simulink model "ModelWithApproximation_20210821T210314460"  (R2020a)
settings: Solver=FixedStepAuto  StartTime=0.0  StopTime=size(InputValues_20210821T203440345,1) - 1  FixedStep=1  RelTol=1e-3
model workspace (MAT data in the model file):
  InputValues_20210821T203440345 = [-1 -0.9921875 -0.984375 -0.9765625 -0.96875 -0.9609375 -0.953125 -0.9453125 -0.9375 -0.9296875 -0.921875 -0.9140625 ... (256 elements, 256x1)]
undefined symbols (not defined in the file or in its folder): FunctionApproximation
libraries: simulink x1
settings Model: OrderedModelArguments=off  Creator=Mahsa  LastModifiedBy=Mahsa
settings DebuggingCC: IntegerOverflowMsg=none  ParameterOverflowMsg=none  ParameterPrecisionLossMsg=none  IntegerSaturationMsg=none

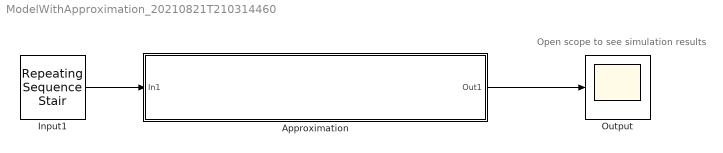
== system ModelWithApproximation_20210821T210314460 ==
  note: Open scope to see simulation results
  Approximation : Subsystem  Description=This block was created using function approximation.  Variant=on  mask(Function Approximation Solution){variantTag=119b4c483346d2625863553620acd5dc80d8d358, createdBy=FunctionApproximation, currentActive=Approximate, nApproximates=1, createdOn=20210821T210309766, matlabVersion={"Name":"MATLAB","Version":"9.8","Release":"(R2020a)","Date":"18-Nov-2019"}, functionVersion=Approximate, problemStruct={"FunctionToApproximate":"@(x)tanh(x)","InputTypes":"numerictype(1,8,7)","InputLowerBounds":"-1","InputUpperBounds":"0.9921875","OutputType":"numerictype(1,8,7)","Options":{"WordLengths":"[8]","BreakpointSpecification":"EvenSpacing","AbsTol":"0.0078125","RelTol":"0.0078125","AllowUpdateDiagram":"1","Display":"1","Interpolation":"Linear","SaturateToOutputType":"0","MaxTime":"Inf","MaxMemoryUsage":"80000000","MemoryUnits":"bits","OnCurveTableValues":"0","AUTOSARCompliant":"0","UseParallel":"0"},"FunctionToReplace":"","InputFunctionType":"SpecialFunctionHandle","StorageTypes":[],"DependentVariables":[]}, compareData={"Breakpoints":[[-1,-0.9921875,-0.984375,-0.9765625,-0.96875,-0.9609375,-0.953125,-0.9453125,-0.9375,-0.9296875,-0.921875,-0.9140625,-0.90625,-0.8984375,-0.890625,-0.8828125,-0.875,-0.8671875,-0.859375,-0.8515625,-0.84375,-0.8359375,-0.828125,-0.8203125,-0.8125,-0.8046875,-0.796875,-0.7890625,-0.78125,-0.7734375,-0.765625,-0.7578125,-0.75,-0.7421875,-0.734375,-0.7265625,-0.71875,-0.7109375,-0.703125,-0.6953125,-0.6875,-0.6796875,-0.671875,-0.6640625,-0.65625,-0.6484375,-0.640625,-0.6328125,-0.625,-0.6171875,-0.609375,-0.6015625,-0.59375,-0.5859375,-0.578125,-0.5703125,-0.5625,-0.5546875,-0.546875,-0.5390625,-0.53125,-0.5234375,-0.515625,-0.5078125,-0.5,-0.4921875,-0.484375,-0.4765625,-0.46875,-0.4609375,-0.453125,-0.4453125,-0.4375,-0.4296875,-0.421875,-0.4140625,-0.40625,-0.3984375,-0.390625,-0.3828125,-0.375,-0.3671875,-0.359375,-0.3515625,-0.34375,-0.3359375,-0.328125,-0.3203125,-0.3125,-0.3046875,-0.296875,-0.2890625,-0.28125,-0.2734375,-0.265625,-0.2578125,-0.25,-0.2421875,-0.234375,-0.2265625,-0.21875,-0.2109375,-0.203125,-0.1953125,-0.1875,-0.1796875,-0.171875,-0.1640625,-0.15625,-0.1484375,-0.140625,-0.1328125,-0.125,-0.1171875,-0.109375,-0.1015625,-0.09375,-0.0859375,-0.078125,-0.0703125,-0.0625,-0.0546875,-0.046875,-0.0390625,-0.03125,-0.0234375,-0.015625,-0.0078125,0,0.0078125,0.015625,0.0234375,0.03125,0.0390625,0.046875,0.0546875,0.0625,0.0703125,0.078125,0.0859375,0.09375,0.1015625,0.109375,0.1171875,0.125,0.1328125,0.140625,0.1484375,0.15625,0.1640625,0.171875,0.1796875,0.1875,0.1953125,0.203125,0.2109375,0.21875,0.2265625,0.234375,0.2421875,0.25,0.2578125,0.265625,0.2734375,0.28125,0.2890625,0.296875,0.3046875,0.3125,0.3203125,0.328125,0.3359375,0.34375,0.3515625,0.359375,0.3671875,0.375,0.3828125,0.390625,0.3984375,0.40625,0.4140625,0.421875,0.4296875,0.4375,0.4453125,0.453125,0.4609375,0.46875,0.4765625,0.484375,0.4921875,0.5,0.5078125,0.515625,0.5234375,0.53125,0.5390625,0.546875,0.5546875,0.5625,0.5703125,0.578125,0.5859375,0.59375,0.6015625,0.609375,0.6171875,0.625,0.6328125,0.640625,0.6484375,0.65625,0.6640625,0.671875,0.6796875,0.6875,0.6953125,0.703125,0.7109375,0.71875,0.7265625,0.734375,0.7421875,0.75,0.7578125,0.765625,0.7734375,0.78125,0.7890625,0.796875,0.8046875,0.8125,0.8203125,0.828125,0.8359375,0.84375,0.8515625,0.859375,0.8671875,0.875,0.8828125,0.890625,0.8984375,0.90625,0.9140625,0.921875,0.9296875,0.9375,0.9453125,0.953125,0.9609375,0.96875,0.9765625,0.984375,0.9921875]],"Original":[-0.76159415595576485,-0.75829353501905861,-0.75495357496368154,-0.7515739832958932,-0.74815447032973548,-0.74469474935641866,-0.74119453681672176,-0.73765355247636877,-0.73407151960434158,-0.73044816515408639,-0.72678321994756123,-0.7230764188620713,-0.71932750101983345,-0.71553620998020728,-0.71170229393451878,-0.70782550590340865,-0.70390560393662116,-0.69994235131514981,-0.69593551675565146,-0.69188487461702919,-0.68779020510908528,-0.68365129450313655,-0.67946793534447858,-0.67523992666657839,-0.67096707420687374,-0.66664919062404671,-0.66228609571663366,-0.65787761664283118,-0.65342358814134682,-0.64892385275314135,-0.644378261043901,-0.63978667182707216,-0.6351489523872873,-0.63046497870399987,-0.62573463567514687,-0.62095781734064481,-0.61613442710552646,-0.61126437796251065,-0.60634759271380312,-0.60138400419190874,-0.59637355547924231,-0.59131620012630826,-0.58621190236822385,-0.58106063733934943,-0.57586239128578931,-0.57061716177551614,-0.56532495790587511,-0.55998580050821367,-0.55459972234938226,-0.54916676832984668,-0.54368699567814927,-0.5381604741414564,-0.53258728617191942,-0.52696752710858485,-0.52130130535457664,-0.515588742549281,-0.50982997373525663,-0.50402514751959449,-0.49817442622945507,-0.49227798606150219,-0.48633601722496222,-0.48034872407803259,-0.47431632525736678,-0.46823905380036612,-0.46211715726000974,-0.455950897811955,-0.44974055235364957,-0.44348641259519572,-0.43718878514171228,-0.43084799156694659,-0.42446436847789382,-0.41803826757018642,-0.41157005567402238,-0.40506011479041065,-0.39850884211751691,-0.39191665006690513,-0.38528396626947237,-0.37861123357089205,-0.37189891001638503,-0.36514746882464827,-0.35835739835078595,-0.35152920203809512,-0.34466339835857224,-0.33776052074201712,-0.330821117493628,-0.32384575169998836,-0.31683500112336604,-0.30978945808425512,-0.30270972933210849,-0.29559643590422069,-0.28845021297273932,-0.28127170967979609,-0.27406158896076638,-0.26682052735568029,-0.25954921480882681,-0.25224835445660676,-0.24491866240370913,-0.23756086748770011,-0.23017571103213297,-0.22276394658830215,-0.21532633966578324,-0.20786366745191662,-0.20037671852040995,-0.19286629252925089,-0.18533319990813948,-0.177778261535664,-0.17020230840646236,-0.16260618128862667,-0.1549907303716235,-0.14735681490501934,-0.1397053028283142,-0.13203707039220292,-0.12435300177159619,-0.11665398867074886,-0.10894092992085458,-0.10121473107048072,-0.093476303969227736,-0.0857265663450104,-0.077966441375368178,-0.070196857253223069,-0.062418746747512514,-0.054633046759134309,-0.046840697872648072,-0.039042643904185916,-0.031239831446031256,-0.023433209408330664,-0.015623728558408866,-0.0078123410581610138,0,0.0078123410581610138,0.015623728558408866,0.023433209408330664,0.031239831446031256,0.039042643904185916,0.046840697872648072,0.054633046759134309,0.062418746747512514,0.070196857253223069,0.077966441375368178,0.0857265663450104,0.093476303969227736,0.10121473107048072,0.10894092992085458,0.11665398867074886,0.12435300177159619,0.13203707039220292,0.1397053028283142,0.14735681490501934,0.1549907303716235,0.16260618128862667,0.17020230840646236,0.177778261535664,0.18533319990813948,0.19286629252925089,0.20037671852040995,0.20786366745191662,0.21532633966578324,0.22276394658830215,0.23017571103213297,0.23756086748770011,0.24491866240370913,0.25224835445660676,0.25954921480882681,0.26682052735568029,0.27406158896076638,0.28127170967979609,0.28845021297273932,0.29559643590422069,0.30270972933210849,0.30978945808425512,0.31683500112336604,0.32384575169998836,0.330821117493628,0.33776052074201712,0.34466339835857224,0.35152920203809512,0.35835739835078595,0.36514746882464827,0.37189891001638503,0.37861123357089205,0.38528396626947237,0.39191665006690513,0.39850884211751691,0.40506011479041065,0.41157005567402238,0.41803826757018642,0.42446436847789382,0.43084799156694659,0.43718878514171228,0.44348641259519572,0.44974055235364957,0.455950897811955,0.46211715726000974,0.46823905380036612 ...(+1232 chars)],"Approximate":[-0.7578125,-0.7578125,-0.7578125,-0.7578125,-0.75,-0.75,-0.7421875,-0.7421875,-0.734375,-0.734375,-0.7265625,-0.7265625,-0.71875,-0.71875,-0.7109375,-0.7109375,-0.703125,-0.703125,-0.6953125,-0.6953125,-0.6875,-0.6875,-0.6796875,-0.6796875,-0.671875,-0.671875,-0.6640625,-0.6640625,-0.65625,-0.6484375,-0.640625,-0.640625,-0.6328125,-0.6328125,-0.625,-0.625,-0.6171875,-0.6171875,-0.609375,-0.6015625,-0.59375,-0.59375,-0.5859375,-0.5859375,-0.578125,-0.5703125,-0.5625,-0.5625,-0.5546875,-0.5546875,-0.546875,-0.5390625,-0.53125,-0.53125,-0.5234375,-0.515625,-0.5078125,-0.5078125,-0.5,-0.4921875,-0.484375,-0.484375,-0.4765625,-0.46875,-0.4609375,-0.4609375,-0.453125,-0.4453125,-0.4375,-0.4296875,-0.421875,-0.421875,-0.4140625,-0.40625,-0.3984375,-0.390625,-0.3828125,-0.3828125,-0.375,-0.3671875,-0.359375,-0.3515625,-0.34375,-0.3359375,-0.328125,-0.328125,-0.3203125,-0.3125,-0.3046875,-0.296875,-0.2890625,-0.28125,-0.2734375,-0.265625,-0.2578125,-0.25,-0.2421875,-0.234375,-0.2265625,-0.2265625,-0.21875,-0.2109375,-0.203125,-0.1953125,-0.1875,-0.1796875,-0.171875,-0.1640625,-0.15625,-0.1484375,-0.140625,-0.1328125,-0.125,-0.1171875,-0.109375,-0.1015625,-0.09375,-0.0859375,-0.078125,-0.0703125,-0.0625,-0.0546875,-0.046875,-0.0390625,-0.03125,-0.0234375,-0.015625,-0.0078125,0,0.0078125,0.015625,0.0234375,0.03125,0.0390625,0.046875,0.0546875,0.0625,0.0703125,0.078125,0.0859375,0.09375,0.1015625,0.109375,0.1171875,0.125,0.1328125,0.140625,0.1484375,0.15625,0.1640625,0.171875,0.1796875,0.1875,0.1953125,0.203125,0.2109375,0.21875,0.21875,0.2265625,0.234375,0.2421875,0.25,0.2578125,0.265625,0.2734375,0.28125,0.2890625,0.296875,0.3046875,0.3125,0.3203125,0.3203125,0.328125,0.3359375,0.34375,0.3515625,0.359375,0.3671875,0.375,0.375,0.3828125,0.390625,0.3984375,0.40625,0.4140625,0.4140625,0.421875,0.4296875,0.4375,0.4453125,0.453125,0.453125,0.4609375,0.46875,0.4765625,0.4765625,0.484375,0.4921875,0.5,0.5,0.5078125,0.515625,0.5234375,0.5234375,0.53125,0.5390625,0.546875,0.546875,0.5546875,0.5546875,0.5625,0.5703125,0.578125,0.578125,0.5859375,0.5859375,0.59375,0.6015625,0.609375,0.609375,0.6171875,0.6171875,0.625,0.625,0.6328125,0.6328125,0.640625,0.6484375,0.65625,0.65625,0.6640625,0.6640625,0.671875,0.671875,0.6796875,0.6796875,0.6875,0.6875,0.6953125,0.6953125,0.703125,0.703125,0.7109375,0.7109375,0.71875,0.71875,0.7265625,0.7265625,0.734375,0.734375,0.7421875,0.7421875,0.75,0.75,0.7578125,0.7578125],"AbsDiff":[0.003781655955764851,0.00048103501905860657,0.0028589250363184604,0.0062385167041068,0.001845529670264523,0.0053052506435813385,0.00099296318327823929,0.0045339475236312321,0.00030348039565841756,0.0039268348459136071,0.00022071994756123203,0.0034860811379286982,0.00057750101983344848,0.0032137900197927172,0.00076479393451878153,0.0031119940965913528,0.00078060393662116034,0.0031826486848501867,0.00062301675565146208,0.0034276253829708114,0.00029020510908528419,0.0038487054968634471,0.00021956465552142035,0.0044475733334216061,0.000907925793126263,0.0052258093759532942,0.0017764042833663396,0.0061848833571688244,0.0028264118586531772,0.00048635275314135029,0.0037532610439009462,0.000838328172927838,0.0023364523872873022,0.0023475212960001324,0.00073463567514686634,0.0040421826593551868,0.001053072894473539,0.0059231220374893478,0.0030274072861968815,0.00017849580809126131,0.0026235554792423121,0.0024337998736917443,0.00027440236822384723,0.0048768626606505716,0.00226260871421069,0.00030466177551613516,0.002824957905875114,0.0025141994917863286,8.7777650617737457E-5,0.0055207316701533227,0.0031880043218507348,0.00090202585854359807,0.0013372861719194162,0.0042824728914151455,0.0021361946454233616,3.625745071900166E-5,0.0020174737352566252,0.0037873524804055148,0.0018255737705449304,9.048606150219296E-5,0.0019610172249622249,0.0040262759219674149,0.0022461747426332224,0.00051094619963387711,0.0011796572600097366,0.0049866021880449751,0.0033844476463504303,0.0018260874048042774,0.00031121485828772277,0.0011604915669465865,0.0025893684778938164,0.003836732429813583,0.0024924443259776163,0.0011898852095893475,7.1342117516914882E-5,0.0012916500669051256,0.0024714662694723666,0.0042012664291079527,0.0031010899836149686,0.0020400311753517308,0.0010176016492140505,3.3297961904876772E-5,0.00091339835857223717,0.0018230207420171229,0.0026961174936280252,0.00427924830001164,0.0034774988766339554,0.0027105419157448796,0.0019777706678915097,0.001278564095779311,0.00061228702726068285,2.1709679796089176E-5,0.000624088960766378,0.0011955273556802926,0.0017367148088268114,0.0022483544566067604,0.0027311624037091309,0.0031858674877001114,0.003613211032132968,0.0037985534116978525,0.0034236603342167604,0.0030738325480833828,0.0027482814795900534,0.0024462074707491122,0.0021668000918605157,0.0019092384643359939,0.0016726915935376396,0.0014563187113733334,0.001259269628376497,0.0010806850949806601,0.00091969717168580156,0.00077542960779708459,0.00064699822840380561,0.00053351132925114064,0.00043407007914542106,0.00034776892951927929,0.00027369603077226357,0.00021093365498960071,0.00015855862463182158,0.00011564274677693109,8.1253252487485661E-5,5.4453240865691421E-5,3.4302127351927558E-5,1.9856095814084485E-5,1.0168553968743776E-5,4.2905916693355972E-6,1.2714415911340565E-6,1.5894183898624431E-7,0,1.5894183898624431E-7,1.2714415911340565E-6,4.2905916693355972E-6,1.0168553968743776E-5,1.9856095814084485E-5,3.4302127351927558E-5,5.4453240865691421E-5,8.1253252487485661E-5,0.00011564274677693109,0.00015855862463182158,0.00021093365498960071,0.00027369603077226357,0.00034776892951927929,0.00043407007914542106,0.00053351132925114064,0.00064699822840380561,0.00077542960779708459,0.00091969717168580156,0.0010806850949806601,0.001259269628376497,0.0014563187113733334,0.0016726915935376396,0.0019092384643359939,0.0021668000918605157,0.0024462074707491122,0.0027482814795900534,0.0030738325480833828,0.0034236603342167604,0.0040139465883021475,0.003613211032132968,0.0031858674877001114,0.0027311624037091309,0.0022483544566067604,0.0017367148088268114,0.0011955273556802926,0.000624088960766378,2.1709679796089176E-5,0.00061228702726068285,0.001278564095779311,0.0019777706678915097,0.0027105419157448796,0.0034774988766339554,0.00353325169998836,0.0026961174936280252,0.0018230207420171229,0.00091339835857223717,3.3297961904876772E-5,0.0010176016492140505,0.0020400311753517308,0.0031010899836149686,0.0036112335708920473,0.0024714662694723666 ...(+1658 chars)],"MaxDiff":[0.0078125,0.0078125,0.0078125,0.0078125,0.0078125,0.0078125,0.0078125,0.0078125,0.0078125,0.0078125,0.0078125,0.0078125,0.0078125,0.0078125,0.0078125,0.0078125,0.0078125,0.0078125,0.0078125,0.0078125,0.0078125,0.0078125,0.0078125,0.0078125,0.0078125,0.0078125,0.0078125,0.0078125,0.0078125,0.0078125,0.0078125,0.0078125,0.0078125,0.0078125,0.0078125,0.0078125,0.0078125,0.0078125,0.0078125,0.0078125,0.0078125,0.0078125,0.0078125,0.0078125,0.0078125,0.0078125,0.0078125,0.0078125,0.0078125,0.0078125,0.0078125,0.0078125,0.0078125,0.0078125,0.0078125,0.0078125,0.0078125,0.0078125,0.0078125,0.0078125,0.0078125,0.0078125,0.0078125,0.0078125,0.0078125,0.0078125,0.0078125,0.0078125,0.0078125,0.0078125,0.0078125,0.0078125,0.0078125,0.0078125,0.0078125,0.0078125,0.0078125,0.0078125,0.0078125,0.0078125,0.0078125,0.0078125,0.0078125,0.0078125,0.0078125,0.0078125,0.0078125,0.0078125,0.0078125,0.0078125,0.0078125,0.0078125,0.0078125,0.0078125,0.0078125,0.0078125,0.0078125,0.0078125,0.0078125,0.0078125,0.0078125,0.0078125,0.0078125,0.0078125,0.0078125,0.0078125,0.0078125,0.0078125,0.0078125,0.0078125,0.0078125,0.0078125,0.0078125,0.0078125,0.0078125,0.0078125,0.0078125,0.0078125,0.0078125,0.0078125,0.0078125,0.0078125,0.0078125,0.0078125,0.0078125,0.0078125,0.0078125,0.0078125,0.0078125,0.0078125,0.0078125,0.0078125,0.0078125,0.0078125,0.0078125,0.0078125,0.0078125,0.0078125,0.0078125,0.0078125,0.0078125,0.0078125,0.0078125,0.0078125,0.0078125,0.0078125,0.0078125,0.0078125,0.0078125,0.0078125,0.0078125,0.0078125,0.0078125,0.0078125,0.0078125,0.0078125,0.0078125,0.0078125,0.0078125,0.0078125,0.0078125,0.0078125,0.0078125,0.0078125,0.0078125,0.0078125,0.0078125,0.0078125,0.0078125,0.0078125,0.0078125,0.0078125,0.0078125,0.0078125,0.0078125,0.0078125,0.0078125,0.0078125,0.0078125,0.0078125,0.0078125,0.0078125,0.0078125,0.0078125,0.0078125,0.0078125,0.0078125,0.0078125,0.0078125,0.0078125,0.0078125,0.0078125,0.0078125,0.0078125,0.0078125,0.0078125,0.0078125,0.0078125,0.0078125,0.0078125,0.0078125,0.0078125,0.0078125,0.0078125,0.0078125,0.0078125,0.0078125,0.0078125,0.0078125,0.0078125,0.0078125,0.0078125,0.0078125,0.0078125,0.0078125,0.0078125,0.0078125,0.0078125,0.0078125,0.0078125,0.0078125,0.0078125,0.0078125,0.0078125,0.0078125,0.0078125,0.0078125,0.0078125,0.0078125,0.0078125,0.0078125,0.0078125,0.0078125,0.0078125,0.0078125,0.0078125,0.0078125,0.0078125,0.0078125,0.0078125,0.0078125,0.0078125,0.0078125,0.0078125,0.0078125,0.0078125,0.0078125,0.0078125,0.0078125,0.0078125,0.0078125,0.0078125,0.0078125,0.0078125,0.0078125,0.0078125],"Feasible":true,"Options":{"WordLengths":8,"BreakpointSpecification":"EvenSpacing","AbsTol":0.0078125,"RelTol":0.0078125,"AllowUpdateDiagram":true,"Display":true,"Interpolation":"Linear","SaturateToOutputType":false,"MaxTime":null,"MaxMemoryUsage":8.0E+7,"MemoryUnits":"bits","OnCurveTableValues":false,"AUTOSARCompliant":false,"UseParallel":false}}}
      mask prompts: functionVersion "Select desired function version"
      mask help: This block contains the original and approximate functions.
      settings: CopyFcn=FunctionApproximation.internal.approximationblock.callback.updateTag('119b4c483346d2625863553620acd5dc80d8d358');  OpenFcn=FunctionApproximation.internal.approximationblock.callback.openMask('119b4c483346d2625863553620acd5dc80d8d358');
      mask Help: helpview(fullfile(docroot,'fixedpoint','fixedpoint.map'), 'function_approximation_block')
      mask TypeOptions functionVersion: Original | Approximate
      mask Callback functionVersion: FunctionApproximation.internal.approximationblock.callback.registerActiveFunction('119b4c483346d2625863553620acd5dc80d8d358');
      mask DialogControl details Prompt: Problem Definition
      mask DialogControl details Tooltip: Details of problem definition for approximation
      mask DialogControl detailsText Prompt:
      | Inputs for approximation:
      |   InputLowerBounds: -1
      |   InputTypes: numerictype(1,8,7)
      |   InputUpperBounds: 0.9921875
      |   OutputType: numerictype(1,8,7)
      |   Options (non-default)
      |     AbsTol: 0.0078125
      |     BreakpointSpecification: EvenSpacing
      |     OnCurveTableValues: 0
      |     RelTol: 0.0078125
      |     WordLengths: [8]
      mask DialogControl showOriginal Prompt: Show original
      mask DialogControl showOriginal Tooltip: View the original function
      mask DialogControl showOriginal Callback: FunctionApproximation.internal.approximationblock.callback.showFunction('119b4c483346d2625863553620acd5dc80d8d358','Original');
      mask DialogControl showCurrent Prompt: Show selected
      mask DialogControl showCurrent Tooltip: View the selected function
      mask DialogControl showCurrent Callback: FunctionApproximation.internal.approximationblock.callback.showCurrent('119b4c483346d2625863553620acd5dc80d8d358');
      mask DialogControl revertToOriginal Prompt: Replace with original
      mask DialogControl revertToOriginal Tooltip: Replace current block with the original function
      mask DialogControl revertToOriginal Callback: FunctionApproximation.internal.approximationblock.callback.revertDialog('119b4c483346d2625863553620acd5dc80d8d358');
      mask DialogControl redesign Prompt: Redesign approximate
      mask DialogControl redesign Tooltip: Obtain a new approximate for the original function.
      mask DialogControl redesign Callback: FunctionApproximation.internal.approximationblock.callback.redesign('119b4c483346d2625863553620acd5dc80d8d358');
      mask DialogControl compare Prompt: Compare to original
      mask DialogControl compare Tooltip: Visualize difference between original and selected function.
      mask DialogControl compare Callback: FunctionApproximation.internal.approximationblock.callback.compareToOriginal('119b4c483346d2625863553620acd5dc80d8d358');
  Input1 : simulink/Sources/Repeating Sequence Stair  OutValues=InputValues_20210821T203440345(:,1)  tsamp=-1  OutMin=[]  OutMax=[]  OutDataTypeStr=fixdt(1,16)  OutputDataTypeScalingMode=Specify via dialog  OutDataType=fixdt(1,16)  ConRadixGroup=Best Precision: Vector-wise  OutScaling=[]
  Output : Scope
  wires:
  Input1/1 -> Approximation/1(In1)
  Approximation/1(Out1) -> Output/1

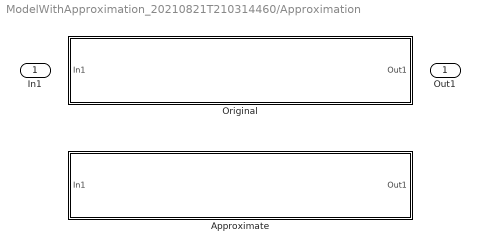
== system ModelWithApproximation_20210821T210314460/Approximation ==
  In1 : Inport
  Approximate : Subsystem  Tag=Approximate  VariantControl=FunctionApproximation.internal.approximationblock.callback.isCurrent('119b4c483346d2625863553620acd5dc80d8d358','Approximate')
  Original : Subsystem  Tag=Original  VariantControl=FunctionApproximation.internal.approximationblock.callback.isCurrent('119b4c483346d2625863553620acd5dc80d8d358','Original')
  Out1 : Outport

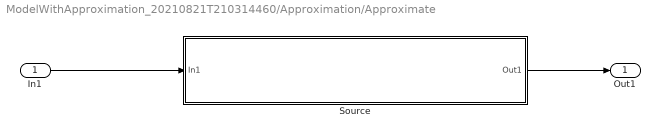
== system ModelWithApproximation_20210821T210314460/Approximation/Approximate ==
  In1 : Inport
  Source : Subsystem  Description=This block was created using function approximation.
  Out1 : Outport
  wires:
  In1/1 -> Source/1(In1)
  Source/1(Out1) -> Out1/1

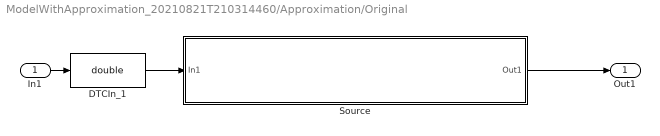
== system ModelWithApproximation_20210821T210314460/Approximation/Original ==
  In1 : Inport
  DTCIn_1 : DataTypeConversion  OutDataTypeStr=double  RndMeth=Nearest
  Source : Subsystem
      mask Display: fprintf('%s','tanh')
  Out1 : Outport
  wires:
  In1/1 -> DTCIn_1/1
  DTCIn_1/1 -> Source/1(In1)
  Source/1(Out1) -> Out1/1

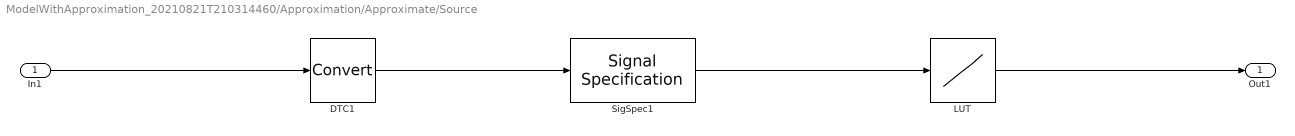
== system ModelWithApproximation_20210821T210314460/Approximation/Approximate/Source ==
  In1 : Inport
  DTC1 : DataTypeConversion  RndMeth=Nearest
  LUT : Lookup_n-D  NumberOfTableDimensions=1  LookupTableObject=FunctionApproximation_LUTObject_20210821T203440330  BreakpointsSpecification=Even spacing  BreakpointsForDimension3=[5, 7]  BreakpointsForDimension1FirstPoint=-1  BreakpointsForDimension1Spacing=0.015625  BreakpointsForDimension1DataTypeStr=numerictype(1,8,7)  IndexSearchMethod=Evenly spaced points  Table=[-0.7578125 -0.7578125 -0.75 -0.7421875 -0.734375 -0.7265625 -0.71875 -0.7109375 -0.703125 -0.6953125 -0.6875 -0.6796875 -0.671875 -0.6640625 -0.65625 -0.640625 -0.6328125 -0.625 -0.6171875 -0.609375 -0.59375 -0.5859375 -0.578125 -0.5625 -0.5546875 -0.546875 -0.53125 -0.5234375 -0.5078125 -0.5 -0.484375 -0.4765625 -0.4609375 -0.453125 -0.4375 -0.421875 -0.4140625 -0.3984375 -0.3828125 -0.375 -0.359375 -0.34375 -0.328125 -0.3203125 -0.3046875 -0.2890625 -0.2734375 -0.2578125 -0.2421875 -0.2265625 -0.21875 -0.203125 -0.1875 -0.171875 -0.15625 -0.140625 -0.125 -0.109375 -0.09375 -0.078125 -0.0625 -0.046875 -0.03125 -0.015625 0 0.015625 0.03125 0.046875 0.0625 0.078125 0.09375 0.109375 0.125 0.140625 0.15625 0.171875 0.1875 0.203125 0.21875 0.2265625 0.2421875 0.2578125 0.2734375 0.2890625 0.3046875 0.3203125 0.328125 0.34375 0.359375 0.375 0.3828125 0.3984375 0.4140625 0.421875 0.4375 0.453125 0.4609375 0.4765625 0.484375 0.5 0.5078125 0.5234375 0.53125 0.546875 0.5546875 0.5625 0.578125 0.5859375 0.59375 0.609375 0.6171875 0.625 0.6328125 0.640625 0.65625 0.6640625 0.671875 0.6796875 0.6875 0.6953125 0.703125 0.7109375 0.71875 0.7265625 0.734375 0.7421875 0.75 0.7578125]  TableDataTypeStr=numerictype(1,8,7)  ExtrapMethod=Clip  UseLastTableValue=on  InternalRulePriority=Speed  OutDataTypeStr=numerictype(1,8,7)  RndMeth=Simplest
  SigSpec1 : SignalSpecification  OutMin=-1  OutMax=0.9921875  OutDataTypeStr=numerictype(1,8,7)
  Out1 : Outport
  wires:
  In1/1 -> DTC1/1
  LUT/1 -> Out1/1
  SigSpec1/1 -> LUT/1
  DTC1/1 -> SigSpec1/1

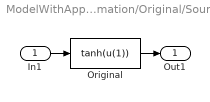
== system ModelWithApproximation_20210821T210314460/Approximation/Original/Source ==
  In1 : Inport
  Original : MATLABFcn  MATLABFcn=tanh(u(1))
  Out1 : Outport
  wires:
  Original/1 -> Out1/1
  In1/1 -> Original/1
